simulink model "SpeedgoatCANOpen2Buses100us"  (R2018b)
settings: Solver=ode8  StartTime=0.0  StopTime=inf  FixedStep=0.0001  RelTol=1e-3  EnableMultiTasking=on
undefined symbols (not defined in the file or in its folder): DiscIntNeverNeededParam
libraries: slrtlib x6, speedgoatlib_IO691 x5, simulink x3, dspstat3 x2
(part 2 of 2)

== system SpeedgoatCANOpen2Buses100us/Speedgoat_TPDOs/CAN Bus Communication/CANOpen Slave Protocol Stack - CAN Bus #2 (B) ==
  C Caller : CCaller  FunctionName=CANOpenSlave_ProcessStack_APT  PortSpecificationStruct="%)30     .    ( D   8    (     @         %    \"     8    !     0         %  0 \"0    $    V    07)G3F%M90  4&]R=$YA;64 4V-O<&4     26YD97@     5'EP90      4VEZ90         .    ,     8    (    !          %    \"     $    $     0         0  0 <GA)1 X    P    !@    @    $          4    (     0    0    !         !  ! !R>$E$#@   #@    &    \"     0         !0    @    !    !0    $         $     4   !);G ...(+2763 chars)"
  CAN RX Wrapper : Subsystem
  CAN TX Wrapper : Subsystem
  wires:
  CAN RX Wrapper/3(DATA) -> C Caller/3
  C Caller/3 -> CAN TX Wrapper/3(DATA)
  CAN RX Wrapper/2(DLC) -> C Caller/2
  C Caller/1 -> CAN TX Wrapper/1(ID)
  CAN RX Wrapper/1(ID) -> C Caller/1
  C Caller/2 -> CAN TX Wrapper/2(DLC), CAN TX Wrapper/Enable

== system SpeedgoatCANOpen2Buses100us/Trike Application Layer/System_Control/BrakeControl ==
  Brake control [%] : Inport
  Amp2mAmp : Gain  Gain=1000
  Data Type Conversion : DataTypeConversion  OutDataTypeStr=uint16
  Gain1 : Gain  Gain=12.7
  Gain2 : Gain  Gain=-1
  Gain3 : Gain  Gain=0.00015625
  Saturation : Saturate  UpperLimit=0  LowerLimit=-1
  Saturation1 : Saturate  UpperLimit=10000  LowerLimit=3600
  Sum : Sum  Inputs=|+-
  offset : Constant  Value=3600
  Br CurrentRef [mA] : Outport
  wires:
  Saturation/1 -> Gain1/1
  Gain1/1 -> Amp2mAmp/1
  Brake control [%]/1 -> Data Type Conversion/1
  Gain2/1 -> Saturation/1
  Amp2mAmp/1 -> Br CurrentRef [mA]/1  "Br CurrentRef"
  Sum/1 -> Gain3/1
  offset/1 -> Sum/2
  Gain3/1 -> Gain2/1  "br_percent"
  Data Type Conversion/1 -> Saturation1/1
  Saturation1/1 -> Sum/1

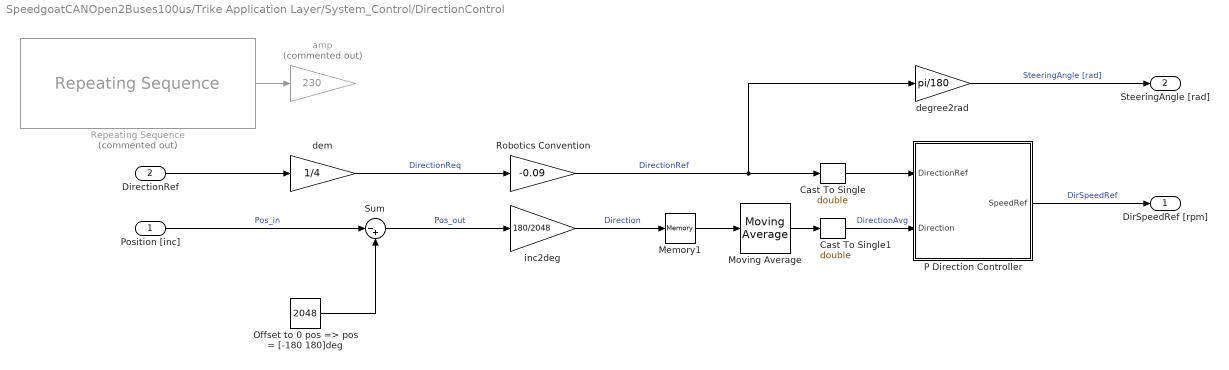
== system SpeedgoatCANOpen2Buses100us/Trike Application Layer/System_Control/DirectionControl ==
  Position [inc] : Inport
  DirectionRef : Inport  Port=2
  Cast To Single : DataTypeConversion  OutDataTypeStr=double
  Cast To Single1 : DataTypeConversion  OutDataTypeStr=double
  Memory1 : Memory  InheritSampleTime=on
  Moving Average : dspstat3/Moving Average  Method=Sliding window  ForgettingFactorPort=off  SpecifyWindowLength=on  WindowLength=1  ForgettingFactor=0.9  SimulateUsing=Code generation
  Offset to 0 pos => pos = [-180 180]deg : Constant  Value=2048
  P Direction Controller : MATLAB Function  TreatAsAtomicUnit=on  SystemSampleTime=5e-3
  Repeating Sequence : simulink/Sources/Repeating Sequence  Commented=on  rep_seq_t=[0 3 3.01 6 6.01 9 9.01 12]*5  rep_seq_y=[1 1 0 0 -1 -1 0 0]
  Robotics Convention : Gain  Gain=-0.09
  Sum : Sum  Inputs=|-+
  amp : Gain  Commented=on  Gain=230
  degree2rad : Gain  Gain=pi/180
  dem : Gain  Gain=1/4
  inc2deg : Gain  Gain=180/2048
  DirSpeedRef [rpm] : Outport
  SteeringAngle [rad] : Outport  Port=2
  wires:
  Memory1/1 -> Moving Average/1
  degree2rad/1 -> SteeringAngle [rad]/1  "SteeringAngle [rad]"
  inc2deg/1 -> Memory1/1  "Direction"
  DirectionRef/1 -> dem/1
  P Direction Controller/1(SpeedRef) -> DirSpeedRef [rpm]/1  "DirSpeedRef"
  Robotics Convention/1 -> Cast To Single/1, degree2rad/1  "DirectionRef"
  Cast To Single/1 -> P Direction Controller/1(DirectionRef)
  Cast To Single1/1 -> P Direction Controller/2(Direction)  "DirectionAvg"
  Position [inc]/1 -> Sum/1  "Pos_in"
  Sum/1 -> inc2deg/1  "Pos_out"
  Offset to 0 pos => pos = [-180 180]deg/1 -> Sum/2
  Moving Average/1 -> Cast To Single1/1
  Repeating Sequence/1 -> amp/1
  dem/1 -> Robotics Convention/1  "DirectionReq"

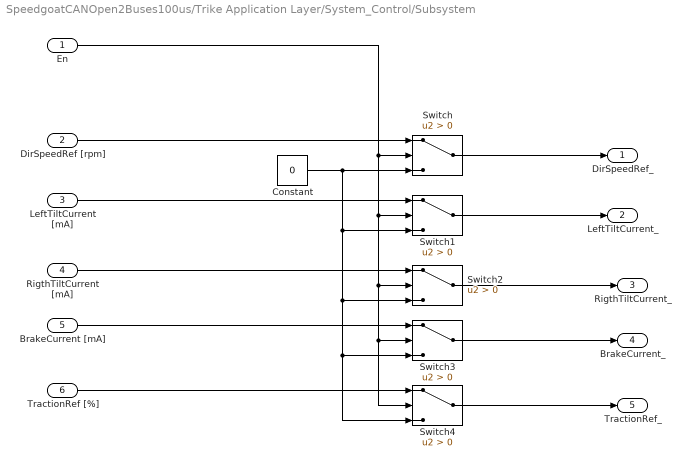
== system SpeedgoatCANOpen2Buses100us/Trike Application Layer/System_Control/Subsystem ==
  En : Inport
  DirSpeedRef [rpm] : Inport  Port=2
  LeftTiltCurrent [mA] : Inport  Port=3
  RigthTiltCurrent [mA] : Inport  Port=4
  BrakeCurrent [mA] : Inport  Port=5
  TractionRef [%] : Inport  Port=6
  Constant : Constant  Value=0
  Switch{,1..4} (5 alike) : Switch  Criteria=u2 > Threshold
  DirSpeedRef_ : Outport
  LeftTiltCurrent_ : Outport  Port=2
  RigthTiltCurrent_ : Outport  Port=3
  BrakeCurrent_ : Outport  Port=4
  TractionRef_ : Outport  Port=5
  wires:
  TractionRef [%]/1 -> Switch4/1
  Switch1/1 -> LeftTiltCurrent_/1
  Switch2/1 -> RigthTiltCurrent_/1
  En/1 -> Switch1/2, Switch2/2, Switch3/2, Switch4/2, Switch/2
  DirSpeedRef [rpm]/1 -> Switch/1
  LeftTiltCurrent [mA]/1 -> Switch1/1
  Constant/1 -> Switch3/3, Switch4/3, Switch2/3, Switch1/3, Switch/3
  Switch/1 -> DirSpeedRef_/1
  BrakeCurrent [mA]/1 -> Switch3/1
  Switch3/1 -> BrakeCurrent_/1
  Switch4/1 -> TractionRef_/1
  RigthTiltCurrent [mA]/1 -> Switch2/1

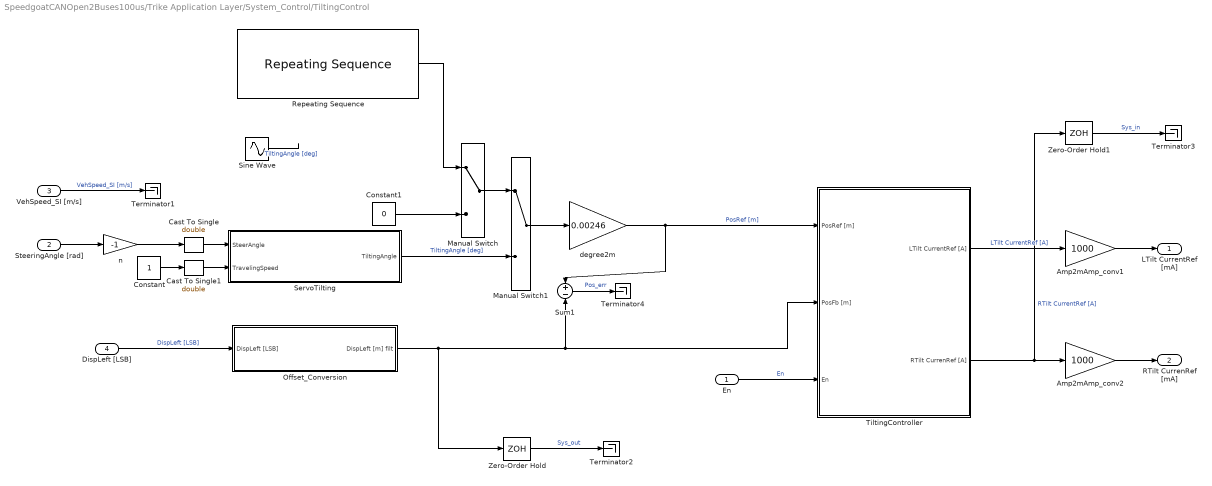
== system SpeedgoatCANOpen2Buses100us/Trike Application Layer/System_Control/TiltingControl ==
  En : Inport
  SteeringAngle [rad] : Inport  Port=2
  VehSpeed_SI [m/s] : Inport  Port=3
  DispLeft [LSB] : Inport  Port=4
  Amp2mAmp_conv1 : Gain  Gain=1000
  Amp2mAmp_conv2 : Gain  Gain=1000
  Cast To Single : DataTypeConversion  OutDataTypeStr=double
  Cast To Single1 : DataTypeConversion  OutDataTypeStr=double
  Constant : Constant
  Constant1 : Constant  Value=0
  Manual Switch : ManualSwitch
  Manual Switch1 : ManualSwitch
  Offset_Conversion : Subsystem
  Repeating Sequence : simulink/Sources/Repeating Sequence  rep_seq_t=[0 3 3.01 6 6.01 9 9.01 12]*5  rep_seq_y=[1 1 0 0 -1 -1 0 0]*2
  ServoTilting : MATLAB Function  TreatAsAtomicUnit=on
      settings: MinAlgLoopOccurrences=on
  Sine Wave : Sin  Frequency=0.5  SampleTime=0
  Sum1 : Sum  Inputs=+|-
  Terminator{1..4} (4 alike) : Terminator
  TiltingController : Subsystem  VariantControlMode=Label  Variant=on  VariantControl=Variant1  LabelModeActiveChoice=V1  PropagateVariantConditions=on
  Zero-Order Hold : ZeroOrderHold  SampleTime=0.001
  Zero-Order Hold1 : ZeroOrderHold  SampleTime=0.001
  degree2m : Gain  Gain=0.00246
  n : Gain  Gain=-1
  LTilt CurrentRef [mA] : Outport
  RTilt CurrenRef [mA] : Outport  Port=2
  wires:
  SteeringAngle [rad]/1 -> n/1
  Constant/1 -> Cast To Single1/1
  Cast To Single/1 -> ServoTilting/1(SteerAngle)
  Cast To Single1/1 -> ServoTilting/2(TravelingSpeed)
  Amp2mAmp_conv1/1 -> LTilt CurrentRef [mA]/1
  Amp2mAmp_conv2/1 -> RTilt CurrenRef [mA]/1
  VehSpeed_SI [m/s]/1 -> Terminator1/1  "VehSpeed_SI [m/s]"
  Constant1/1 -> Manual Switch/2
  ServoTilting/1(TiltingAngle) -> Manual Switch1/2  "TiltingAngle [deg]"
  Manual Switch/1 -> Manual Switch1/1
  Manual Switch1/1 -> degree2m/1
  n/1 -> Cast To Single/1
  degree2m/1 -> Sum1/1, TiltingController/1("PosRef [m] ")  "PosRef [m]"
  Sine Wave/1 -> ?  "TiltingAngle [deg]"
  En/1 -> TiltingController/3("En ")  "En"
  Sum1/1 -> Terminator4/1  "Pos_err"
  TiltingController/1(" LTilt CurrentRef [A]") -> Amp2mAmp_conv1/1  "LTilt CurrentRef [A]"
  TiltingController/2(" RTilt CurrenRef [A]") -> Zero-Order Hold1/1, Amp2mAmp_conv2/1  "RTilt CurrentRef [A]"
  Offset_Conversion/1(DispLeft [m] filt) -> Zero-Order Hold/1, TiltingController/2(PosFb [m]), Sum1/2
  DispLeft [LSB]/1 -> Offset_Conversion/1(DispLeft [LSB])  "DispLeft [LSB]"
  Zero-Order Hold/1 -> Terminator2/1  "Sys_out"
  Zero-Order Hold1/1 -> Terminator3/1  "Sys_in"
  Repeating Sequence/1 -> Manual Switch/1

== system SpeedgoatCANOpen2Buses100us/Trike Application Layer/System_Control/TractionControl ==
  Traction Torque [%] : Inport
  SpeedRear_Fb : Inport  Port=2
  Abs : Abs
  Gain1 : Gain  Gain=1/10
  Gain2 : Gain  Gain=pi/30
  Terminator1 : Terminator
  WheelRadius : Gain  Gain=0.25
  m/s2Km/h : Gain  Gain=3.6
  VehSpeed_SI [m/s] : Outport
  TractionRef [%] : Outport  Port=2
  wires:
  Traction Torque [%]/1 -> Gain1/1
  Abs/1 -> TractionRef [%]/1  "TractionRef"
  WheelRadius/1 -> m/s2Km/h/1, VehSpeed_SI [m/s]/1  "VehSpeed_SI"
  SpeedRear_Fb/1 -> Gain2/1
  Gain2/1 -> WheelRadius/1  "SpeedRear_SI"
  m/s2Km/h/1 -> Terminator1/1  "VehSpeed_Km/h"
  Gain1/1 -> Abs/1

== system SpeedgoatCANOpen2Buses100us/Trike Application Layer/System_Init/Brakes_DunkMotor_Init ==
  Joystick_ButtonStatus : Inport
  DunkD_RPDOs : Inport  Port=2  OutDataTypeStr=Bus: Dunk_RPDOs
  Bus Creator : BusCreator  Inputs=4  OutDataTypeStr=Bus: Dunk_Init_TPDOs
  Bus Selector1 : BusSelector  OutputSignals=DunkD_ActualVelocity
  Cast To Single{,1..3} (4 alike) : DataTypeConversion  OutDataTypeStr=uint8
  Constant : Constant  OutDataTypeStr=single
  DunkD_Brake_Init_CurrentMode : Stateflow chart  TreatAsAtomicUnit=on
  Brakes Motor : Outport  OutDataTypeStr=Bus: Dunk_Init_TPDOs
  Brake InitStatus : Outport  Port=2
  wires:
  DunkD_RPDOs/1 -> Bus Selector1/1
  Bus Creator/1 -> Brakes Motor/1
  Cast To Single1/1 -> Bus Creator/1  "ClearError"
  Cast To Single/1 -> Bus Creator/2  "DeviceMode"
  Cast To Single2/1 -> Bus Creator/3  "BrakeCtrl"
  Cast To Single3/1 -> Bus Creator/4  "PowerEnable"
  DunkD_Brake_Init_CurrentMode/5(InitStatus) -> Brake InitStatus/1
  DunkD_Brake_Init_CurrentMode/1(ClearError) -> Cast To Single1/1
  Joystick_ButtonStatus/1 -> DunkD_Brake_Init_CurrentMode/1(ButtonStatus)
  DunkD_Brake_Init_CurrentMode/2(DeviceMode) -> Cast To Single/1
  DunkD_Brake_Init_CurrentMode/3(BrakeCtrl) -> Cast To Single2/1
  DunkD_Brake_Init_CurrentMode/4(PowerEnable) -> Cast To Single3/1
  Constant/1 -> DunkD_Brake_Init_CurrentMode/2(ReadError)

== system SpeedgoatCANOpen2Buses100us/Trike Application Layer/System_Init/Steering_DunkMotor_Init ==
  Joystick_ButtonStatus : Inport
  DunkA_RPDOs : Inport  Port=2  OutDataTypeStr=Bus: Dunk_RPDOs
  Bus Creator : BusCreator  Inputs=4  OutDataTypeStr=Bus: Dunk_Init_TPDOs
  Bus Selector1 : BusSelector  OutputSignals=DunkA_ActualVelocity
  Cast To Single{,1..3} (4 alike) : DataTypeConversion  OutDataTypeStr=uint8
  Constant : Constant  OutDataTypeStr=single
  DunkA_Steering_Init_SpeedMode : Stateflow chart  TreatAsAtomicUnit=on
  Steering Motor : Outport  OutDataTypeStr=Bus: Dunk_Init_TPDOs
  Steering InitStatus : Outport  Port=2
  wires:
  Bus Creator/1 -> Steering Motor/1
  DunkA_RPDOs/1 -> Bus Selector1/1
  DunkA_Steering_Init_SpeedMode/1(ClearError) -> Cast To Single1/1
  DunkA_Steering_Init_SpeedMode/2(DeviceMode) -> Cast To Single/1
  DunkA_Steering_Init_SpeedMode/3(BrakeCtrl) -> Cast To Single2/1
  DunkA_Steering_Init_SpeedMode/4(PowerEnable) -> Cast To Single3/1
  Joystick_ButtonStatus/1 -> DunkA_Steering_Init_SpeedMode/1(ButtonStatus)
  Constant/1 -> DunkA_Steering_Init_SpeedMode/2(ReadError)
  Cast To Single1/1 -> Bus Creator/1  "ClearError"
  Cast To Single/1 -> Bus Creator/2  "DeviceMode"
  Cast To Single2/1 -> Bus Creator/3  "BrakeCtrl"
  Cast To Single3/1 -> Bus Creator/4  "PowerEnable"
  DunkA_Steering_Init_SpeedMode/5(InitStatus) -> Steering InitStatus/1

== system SpeedgoatCANOpen2Buses100us/Trike Application Layer/System_Init/Subsystem ==
  Steering InitStatus : Inport
  TiltLeft InitStatus : Inport  Port=2
  TiltRight InitStatus : Inport  Port=3
  Brake InitStatus : Inport  Port=4
  MiniMaster_Enable : Inport  Port=5
  Compare To Constant : simulink/Logic and Bit Operations/Compare To Constant  relop===  const=5  OutDataTypeStr=boolean
  Sum : Sum  Inputs=+++++
  EnableControl : Outport
  wires:
  Sum/1 -> Compare To Constant/1
  Brake InitStatus/1 -> Sum/4  "Brake_InitStatus"
  Steering InitStatus/1 -> Sum/1  "Steering_InitStatus"
  TiltRight InitStatus/1 -> Sum/3  "TiltRight_InitStatus"
  TiltLeft InitStatus/1 -> Sum/2  "TiltLeft_InitStatus"
  MiniMaster_Enable/1 -> Sum/5  "MiniMaster_Enable"
  Compare To Constant/1 -> EnableControl/1  "EnableControl"

== system SpeedgoatCANOpen2Buses100us/Trike Application Layer/System_Init/TiltingLeft_DunkMotor_Init ==
  Joystick_ButtonStatus : Inport
  DunkB_RPDOs : Inport  Port=2  OutDataTypeStr=Bus: Dunk_RPDOs
  Bus Creator : BusCreator  Inputs=4  OutDataTypeStr=Bus: Dunk_Init_TPDOs
  Bus Selector1 : BusSelector  OutputSignals=DunkB_ActualVelocity
  Cast To Single{,1..3} (4 alike) : DataTypeConversion  OutDataTypeStr=uint8
  Constant : Constant  OutDataTypeStr=single
  DunkB_TiltLeft_Init_CurrentMode : Stateflow chart  TreatAsAtomicUnit=on
  TiltLeft Motor : Outport  OutDataTypeStr=Bus: Dunk_Init_TPDOs
  TiltLeft InitStatus : Outport  Port=2
  wires:
  DunkB_RPDOs/1 -> Bus Selector1/1
  Bus Creator/1 -> TiltLeft Motor/1
  DunkB_TiltLeft_Init_CurrentMode/5(InitStatus) -> TiltLeft InitStatus/1
  Cast To Single/1 -> Bus Creator/2  "DeviceMode"
  Constant/1 -> DunkB_TiltLeft_Init_CurrentMode/2(ReadError)
  Cast To Single2/1 -> Bus Creator/3  "BrakeCtrl"
  DunkB_TiltLeft_Init_CurrentMode/4(PowerEnable) -> Cast To Single3/1
  DunkB_TiltLeft_Init_CurrentMode/3(BrakeCtrl) -> Cast To Single2/1
  Cast To Single3/1 -> Bus Creator/4  "PowerEnable"
  DunkB_TiltLeft_Init_CurrentMode/2(DeviceMode) -> Cast To Single/1
  Cast To Single1/1 -> Bus Creator/1  "ClearError"
  DunkB_TiltLeft_Init_CurrentMode/1(ClearError) -> Cast To Single1/1
  Joystick_ButtonStatus/1 -> DunkB_TiltLeft_Init_CurrentMode/1(ButtonStatus)

== system SpeedgoatCANOpen2Buses100us/Trike Application Layer/System_Init/TiltingRight_DunkMotor_Init ==
  Joystick_ButtonStatus : Inport
  DunkC_RPDOs : Inport  Port=2  OutDataTypeStr=Bus: Dunk_RPDOs
  Bus Creator : BusCreator  Inputs=4  OutDataTypeStr=Bus: Dunk_Init_TPDOs
  Bus Selector1 : BusSelector  OutputSignals=DunkC_ActualVelocity
  Cast To Single{,1..3} (4 alike) : DataTypeConversion  OutDataTypeStr=uint8
  Constant : Constant  OutDataTypeStr=single
  DunkC_TiltRight_Init_CurrentMode : Stateflow chart  TreatAsAtomicUnit=on
  TiltRight Motor : Outport  OutDataTypeStr=Bus: Dunk_Init_TPDOs
  TiltRight InitStatus : Outport  Port=2
  wires:
  Bus Creator/1 -> TiltRight Motor/1
  DunkC_RPDOs/1 -> Bus Selector1/1
  Cast To Single1/1 -> Bus Creator/1  "ClearError"
  Cast To Single/1 -> Bus Creator/2  "DeviceMode"
  Cast To Single2/1 -> Bus Creator/3  "BrakeCtrl"
  Cast To Single3/1 -> Bus Creator/4  "PowerEnable"
  DunkC_TiltRight_Init_CurrentMode/5(InitStatus) -> TiltRight InitStatus/1
  DunkC_TiltRight_Init_CurrentMode/1(ClearError) -> Cast To Single1/1
  Joystick_ButtonStatus/1 -> DunkC_TiltRight_Init_CurrentMode/1(ButtonStatus)
  DunkC_TiltRight_Init_CurrentMode/2(DeviceMode) -> Cast To Single/1
  DunkC_TiltRight_Init_CurrentMode/3(BrakeCtrl) -> Cast To Single2/1
  DunkC_TiltRight_Init_CurrentMode/4(PowerEnable) -> Cast To Single3/1
  Constant/1 -> DunkC_TiltRight_Init_CurrentMode/2(ReadError)

== system SpeedgoatCANOpen2Buses100us/Speedgoat_TPDOs/CAN Bus Communication/CANOpen Slave Protocol Stack - CAN Bus #1 (A)/CAN RX Wrapper ==
  CAN Read : speedgoatlib_IO691/CAN Read  id=1  ts=Ts  channel=1  messageType=RAW  canType=CAN (HS)  initValues=[691 1 0.0001 0 2 1]
      settings: SourceProductName=Simulink Real-Time: Speedgoat Library
  Constant : Constant  Commented=on  Value=0  OutDataTypeStr=Inherit: Inherit via back propagation
  Switch : Switch  Criteria=u2 > Threshold
  Terminator : Terminator
  Terminator1 : Terminator
  ID : Outport
  DLC : Outport  Port=2
  DATA : Outport  Port=3
  wires:
  CAN Read/4 -> Switch/3
  CAN Read/5 -> Terminator1/1
  Switch/1 -> DLC/1
  CAN Read/2 -> ID/1
  CAN Read/3 -> Switch/2
  CAN Read/6 -> DATA/1
  Constant/1 -> Switch/1
  CAN Read/1 -> Terminator/1

== system SpeedgoatCANOpen2Buses100us/Speedgoat_TPDOs/CAN Bus Communication/CANOpen Slave Protocol Stack - CAN Bus #1 (A)/CAN TX Wrapper ==
  ID : Inport
  DLC : Inport  Port=2
  DATA : Inport  Port=3
  Enable : EnablePort
  CAN Write : speedgoatlib_IO691/CAN Write  id=1  ts=Ts  channel=1  messageType=RAW  enableStatusPort=off  canType=CAN (HS)  initValues=[691 1 0.0001 0 2 1 0]
      settings: SourceProductName=Simulink Real-Time: Speedgoat Library
  Constant : Constant  Value=0  OutDataTypeStr=Inherit: Inherit via back propagation
  wires:
  ID/1 -> CAN Write/1
  DATA/1 -> CAN Write/4
  DLC/1 -> CAN Write/3
  Constant/1 -> CAN Write/2

== system SpeedgoatCANOpen2Buses100us/Speedgoat_TPDOs/CAN Bus Communication/CANOpen Slave Protocol Stack - CAN Bus #2 (B)/CAN RX Wrapper ==
  CAN Read : speedgoatlib_IO691/CAN Read  id=1  ts=Ts  channel=2  messageType=RAW  canType=CAN (HS)  initValues=[691 1 0.0001 1 2 1]
      settings: SourceProductName=Simulink Real-Time: Speedgoat Library
  Constant : Constant  Commented=on  Value=0  OutDataTypeStr=Inherit: Inherit via back propagation
  Switch : Switch  Criteria=u2 > Threshold
  Terminator : Terminator
  Terminator1 : Terminator
  ID : Outport
  DLC : Outport  Port=2
  DATA : Outport  Port=3
  wires:
  CAN Read/1 -> Terminator/1
  Constant/1 -> Switch/1
  CAN Read/6 -> DATA/1
  CAN Read/3 -> Switch/2
  CAN Read/2 -> ID/1
  Switch/1 -> DLC/1
  CAN Read/5 -> Terminator1/1
  CAN Read/4 -> Switch/3

== system SpeedgoatCANOpen2Buses100us/Speedgoat_TPDOs/CAN Bus Communication/CANOpen Slave Protocol Stack - CAN Bus #2 (B)/CAN TX Wrapper ==
  ID : Inport
  DLC : Inport  Port=2
  DATA : Inport  Port=3
  Enable : EnablePort
  CAN Write : speedgoatlib_IO691/CAN Write  id=1  ts=Ts  channel=2  messageType=RAW  enableStatusPort=off  canType=CAN (HS)  initValues=[691 1 0.0001 1 2 1 0]
      settings: SourceProductName=Simulink Real-Time: Speedgoat Library
  Constant : Constant  Value=0  OutDataTypeStr=Inherit: Inherit via back propagation
  wires:
  Constant/1 -> CAN Write/2
  DLC/1 -> CAN Write/3
  DATA/1 -> CAN Write/4
  ID/1 -> CAN Write/1

== system SpeedgoatCANOpen2Buses100us/Trike Application Layer/System_Control/TiltingControl/Offset_Conversion ==
  DispLeft [LSB] : Inport
  Discrete Filter : DiscreteFilter  Numerator=[0.0201 0.0402 0.0201]  Denominator=[1 -1.561 0.6414]  SampleTime=0.005
  LSB2Volt : Gain  Gain=5/16380
  Memory1 : Memory  InheritSampleTime=on
  "Offset for 0 deg (3.5064V -> 57.02mm)" : Constant  Value=3.5064
  Sum : Sum  Inputs=|+-
  Volt2meter : Gain  Gain=0.076/5
  DispLeft [m] filt : Outport
  wires:
  Volt2meter/1 -> Memory1/1, Discrete Filter/1  "DispLeft [m]"
  "Offset for 0 deg (3.5064V -> 57.02mm)"/1 -> Sum/2
  Sum/1 -> Volt2meter/1  "DispLeftOffset [Volt]"
  LSB2Volt/1 -> Sum/1  "DispLeft [Volt]"
  Discrete Filter/1 -> ?
  Memory1/1 -> DispLeft [m] filt/1  "DispLeft [m] filt"
  DispLeft [LSB]/1 -> LSB2Volt/1

== system SpeedgoatCANOpen2Buses100us/Trike Application Layer/System_Control/TiltingControl/TiltingController ==
  "PosRef [m] " : Inport
  PosFb [m] : Inport  Port=2
  "En " : Inport  Port=3
  PID_Adaptiv_V2 : Subsystem  VariantControl=V0
  PID_Clasic_V1 : Subsystem  VariantControl=V1
  PID_Incremental_V1 : Subsystem  VariantControl=V2
  PID_Incremental_V2 : Subsystem  VariantControl=V3
  " LTilt CurrentRef [A]" : Outport
  " RTilt CurrenRef [A]" : Outport  Port=2

== system SpeedgoatCANOpen2Buses100us/Trike Application Layer/System_Control/TiltingControl/TiltingController/PID_Adaptiv_V2 ==
  PosRef [m] : Inport
  PosFb [m] : Inport  Port=2
  En : Inport  Port=3
  PID_ctrl : Subsystem  mask{Kp=800, Ki=400, Kd=0, Ts=0.001, N=1, FF_En=1, Req_lim=10}
      mask prompts: N "FilterOrder"; FF_En "FeedForward En"; Req_lim "Req_sat"
  " LTilt CurrentRef [A]" : Outport
  " RTilt CurrenRef [A]" : Outport  Port=2
  wires:
  PosRef [m]/1 -> PID_ctrl/1(PosRef)
  PosFb [m]/1 -> PID_ctrl/2(PosFb)
  PID_ctrl/1(LTilt CurrentRef [A]) -> " LTilt CurrentRef [A]"/1  "LTilt CurrentRef"
  PID_ctrl/2(RTilt CurrentRef [A]) -> " RTilt CurrenRef [A]"/1  "RTilt CurrenRef"
  En/1 -> PID_ctrl/3(En)

== system SpeedgoatCANOpen2Buses100us/Trike Application Layer/System_Control/TiltingControl/TiltingController/PID_Clasic_V1 ==
  PosRef [m] : Inport
  PosFb [m] : Inport  Port=2
  En : Inport  Port=3
  PID_ctrl : Subsystem  mask{Kp=800, Ki=400, Kd=0, Ts=0.001, N=1, FF_En=1, Req_lim=10}
      mask prompts: N "FilterOrder"; FF_En "FeedForward En"; Req_lim "Req_sat"
  " LTilt CurrentRef [A]" : Outport
  " RTilt CurrenRef [A]" : Outport  Port=2
  wires:
  En/1 -> PID_ctrl/3(En)
  PID_ctrl/2(RTilt CurrentRef [A]) -> " RTilt CurrenRef [A]"/1  "RTilt CurrenRef"
  PID_ctrl/1(LTilt CurrentRef [A]) -> " LTilt CurrentRef [A]"/1  "LTilt CurrentRef"
  PosFb [m]/1 -> PID_ctrl/2(PosFb)
  PosRef [m]/1 -> PID_ctrl/1(PosRef)

== system SpeedgoatCANOpen2Buses100us/Trike Application Layer/System_Control/TiltingControl/TiltingController/PID_Incremental_V1 ==
  PosRef [m] : Inport
  PosFb [m] : Inport  Port=2
  En : Inport  Port=3
  PI_incremental Tilting Controller : MATLAB Function  TreatAsAtomicUnit=on  SystemSampleTime=5e-3
  Terminator1 : Terminator
  Terminator2 : Terminator
  Terminator7 : Terminator
  " LTilt CurrentRef [A]" : Outport
  " RTilt CurrenRef [A]" : Outport  Port=2
  wires:
  En/1 -> PI_incremental Tilting Controller/3(En)
  PI_incremental Tilting Controller/2(RTiltCurrRef) -> " RTilt CurrenRef [A]"/1  "RTilt CurrenRef"
  PI_incremental Tilting Controller/1(LTiltCurrRef) -> " LTilt CurrentRef [A]"/1  "LTilt CurrentRef"
  PosFb [m]/1 -> PI_incremental Tilting Controller/2(Pos)
  PosRef [m]/1 -> PI_incremental Tilting Controller/1(PosRef)
  PI_incremental Tilting Controller/3(up) -> Terminator7/1  "up"
  PI_incremental Tilting Controller/4(ui) -> Terminator1/1  "ui"
  PI_incremental Tilting Controller/5(ud) -> Terminator2/1  "ud"

== system SpeedgoatCANOpen2Buses100us/Trike Application Layer/System_Control/TiltingControl/TiltingController/PID_Incremental_V2 ==
  PosRef [m] : Inport
  PosFb [m] : Inport  Port=2
  En : Inport  Port=3
  MATLAB Function : MATLAB Function  TreatAsAtomicUnit=on  SystemSampleTime=0.005
  Terminator1 : Terminator
  Terminator7 : Terminator
  " LTilt CurrentRef [A]" : Outport
  " RTilt CurrenRef [A]" : Outport  Port=2
  wires:
  PosRef [m]/1 -> MATLAB Function/1(PosRef)
  PosFb [m]/1 -> MATLAB Function/2(Pos)
  MATLAB Function/1(LTiltCurrRef) -> " LTilt CurrentRef [A]"/1  "LTilt CurrentRef"
  MATLAB Function/3(c1) -> Terminator7/1  "c1"
  MATLAB Function/2(RTiltCurrRef) -> " RTilt CurrenRef [A]"/1  "RTilt CurrenRef"
  En/1 -> MATLAB Function/3(En)
  MATLAB Function/4(c2) -> Terminator1/1  "c2"

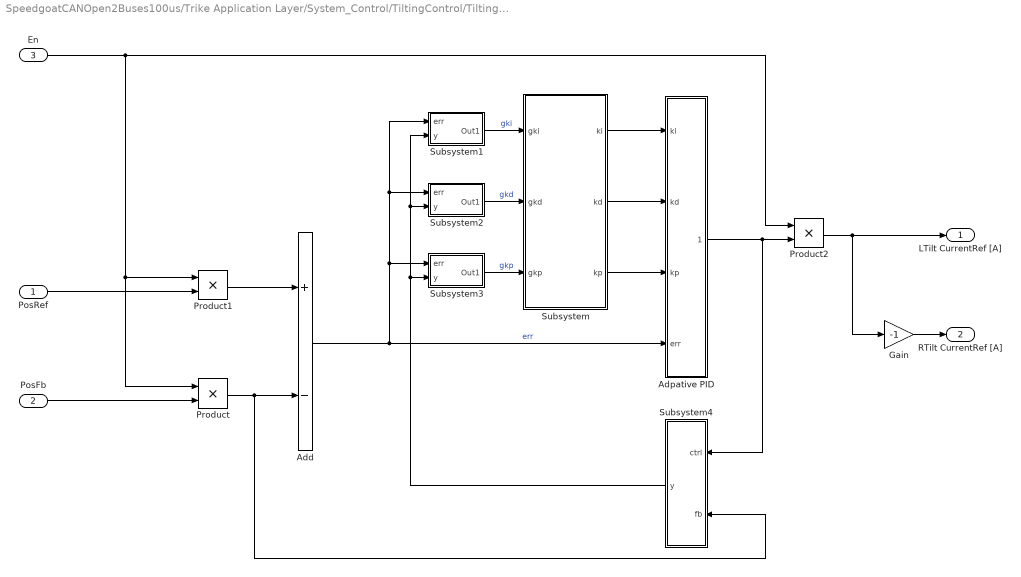
== system SpeedgoatCANOpen2Buses100us/Trike Application Layer/System_Control/TiltingControl/TiltingController/PID_Adaptiv_V2/PID_ctrl ==
  PosRef : Inport
  PosFb : Inport  Port=2
  En : Inport  Port=3
  Add : Sum  Inputs=+-
  Adpative PID : Subsystem
  Gain : Gain  Gain=-1
  Product : Product
  Product1 : Product
  Product2 : Product
  Subsystem : Subsystem
  Subsystem1 : Subsystem
  Subsystem2 : Subsystem
  Subsystem3 : Subsystem
  Subsystem4 : Subsystem
  LTilt CurrentRef [A] : Outport  VectorParamsAs1DForOutWhenUnconnected=on
  RTilt CurrentRef [A] : Outport  Port=2  VectorParamsAs1DForOutWhenUnconnected=on
  wires:
  Gain/1 -> RTilt CurrentRef [A]/1
  Product2/1 -> LTilt CurrentRef [A]/1, Gain/1
  PosRef/1 -> Product1/2
  En/1 -> Product1/1, Product/1, Product2/1
  PosFb/1 -> Product/2
  Subsystem1/1(Out1) -> Subsystem/1(gki)  "gki"
  Subsystem/2(kd) -> Adpative PID/2(kd)
  Subsystem3/1(Out1) -> Subsystem/3(gkp)  "gkp"
  Subsystem/1(ki) -> Adpative PID/1(ki)
  Subsystem/3(kp) -> Adpative PID/3(kp)
  Subsystem2/1(Out1) -> Subsystem/2(gkd)  "gkd"
  Subsystem4/1(y) -> Subsystem3/2(y), Subsystem2/2(y), Subsystem1/2(y)
  Adpative PID/1(ctrl) -> Subsystem4/1(ctrl), Product2/2
  Add/1 -> Subsystem1/1(err), Subsystem2/1(err), Subsystem3/1(err), Adpative PID/4(err)  "err"
  Product1/1 -> Add/1
  Product/1 -> Subsystem4/2(fb), Add/2

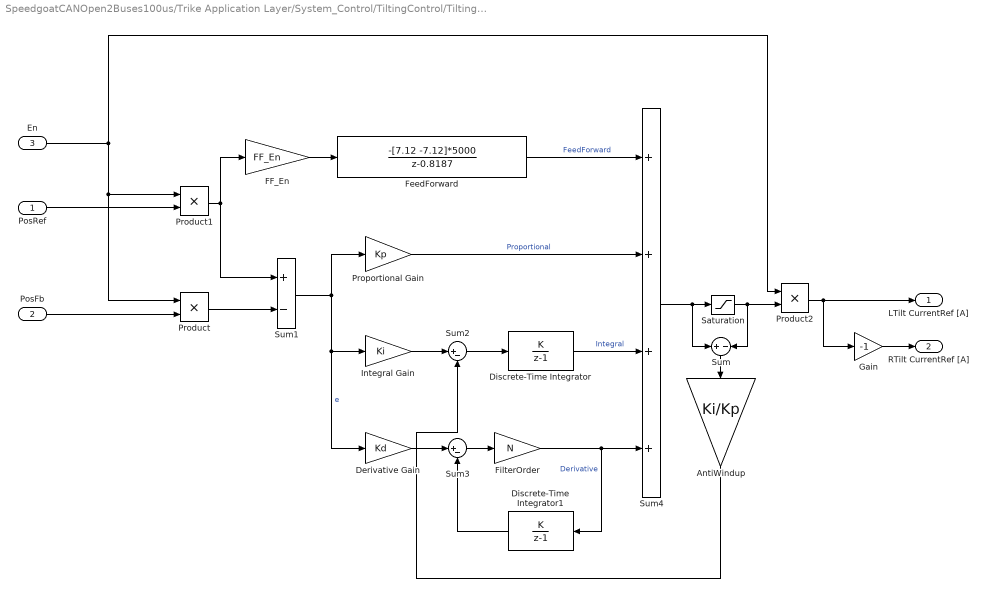
== system SpeedgoatCANOpen2Buses100us/Trike Application Layer/System_Control/TiltingControl/TiltingController/PID_Clasic_V1/PID_ctrl ==
  PosRef : Inport
  PosFb : Inport  Port=2
  En : Inport  Port=3
  AntiWindup : Gain  Gain=Ki/Kp  SaturateOnIntegerOverflow=on  OutDataTypeStr=Inherit: Same as input  ParamDataTypeStr=Inherit: Same as input
  Derivative Gain : Gain  Gain=Kd  SaturateOnIntegerOverflow=on  OutDataTypeStr=Inherit: Same as input  ParamDataTypeStr=Inherit: Same as input
  Discrete-Time Integrator : DiscreteIntegrator  IntegratorMethod=Accumulation: Forward Euler  gainval=Ts/5  SampleTime=-1  ICPrevOutput=DiscIntNeverNeededParam  ICPrevScaledInput=DiscIntNeverNeededParam
  Discrete-Time Integrator1 : DiscreteIntegrator  IntegratorMethod=Accumulation: Forward Euler  gainval=Ts/5  SampleTime=-1  ICPrevOutput=DiscIntNeverNeededParam  ICPrevScaledInput=DiscIntNeverNeededParam
  FF_En : Gain  Gain=FF_En  SaturateOnIntegerOverflow=on  OutDataTypeStr=Inherit: Same as input  ParamDataTypeStr=Inherit: Same as input
  FeedForward : DiscreteTransferFcn  Numerator=-[7.12 -7.12]*5000  Denominator=[1 -0.8187]  SampleTime=Ts/5
  FilterOrder : Gain  Gain=N  SaturateOnIntegerOverflow=on  OutDataTypeStr=Inherit: Same as input  ParamDataTypeStr=Inherit: Same as input
  Gain : Gain  Gain=-1
  Integral Gain : Gain  Gain=Ki  SaturateOnIntegerOverflow=on  OutDataTypeStr=Inherit: Same as input  ParamDataTypeStr=Inherit: Same as input
  Product : Product
  Product1 : Product
  Product2 : Product
  Proportional Gain : Gain  Gain=Kp  SaturateOnIntegerOverflow=on  OutDataTypeStr=Inherit: Same as input  ParamDataTypeStr=Inherit: Same as input
  Saturation : Saturate  UpperLimit=Req_lim  LowerLimit=-Req_lim
  Sum : Sum  Inputs=+|-
  Sum1 : Sum  Inputs=+-  SaturateOnIntegerOverflow=on  InputSameDT=on  OutDataTypeStr=Inherit: Same as first input
  Sum2 : Sum  Inputs=|+-
  Sum3 : Sum  Inputs=|+-
  Sum4 : Sum  Inputs=++++  SaturateOnIntegerOverflow=on  InputSameDT=on  OutDataTypeStr=Inherit: Same as first input
  LTilt CurrentRef [A] : Outport  VectorParamsAs1DForOutWhenUnconnected=on
  RTilt CurrentRef [A] : Outport  Port=2  VectorParamsAs1DForOutWhenUnconnected=on
  wires:
  Saturation/1 -> Product2/2, Sum/2
  AntiWindup/1 -> Sum2/2
  Sum2/1 -> Discrete-Time Integrator/1
  Sum4/1 -> Sum/1, Saturation/1
  FeedForward/1 -> Sum4/1  "FeedForward"
  Proportional Gain/1 -> Sum4/2  "Proportional"
  Integral Gain/1 -> Sum2/1
  Sum/1 -> AntiWindup/1
  Discrete-Time Integrator/1 -> Sum4/3  "Integral"
  PosFb/1 -> Product/2
  Product1/1 -> Sum1/1, FF_En/1
  Product/1 -> Sum1/2
  En/1 -> Product2/1, Product/1, Product1/1
  PosRef/1 -> Product1/2
  Product2/1 -> Gain/1, LTilt CurrentRef [A]/1
  Gain/1 -> RTilt CurrentRef [A]/1
  Derivative Gain/1 -> Sum3/1
  Discrete-Time Integrator1/1 -> Sum3/2
  Sum1/1 -> Proportional Gain/1, Derivative Gain/1, Integral Gain/1  "e"
  Sum3/1 -> FilterOrder/1
  FilterOrder/1 -> Sum4/4, Discrete-Time Integrator1/1  "Derivative"
  FF_En/1 -> FeedForward/1

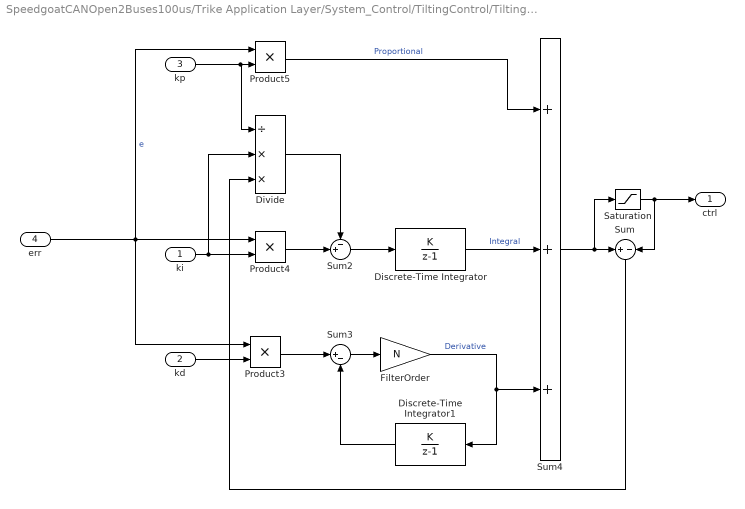
== system SpeedgoatCANOpen2Buses100us/Trike Application Layer/System_Control/TiltingControl/TiltingController/PID_Adaptiv_V2/PID_ctrl/Adpative PID ==
  ki : Inport
  kd : Inport  Port=2
  kp : Inport  Port=3
  err : Inport  Port=4
  Discrete-Time Integrator : DiscreteIntegrator  IntegratorMethod=Accumulation: Forward Euler  gainval=Ts/2  SampleTime=-1  ICPrevOutput=DiscIntNeverNeededParam  ICPrevScaledInput=DiscIntNeverNeededParam
  Discrete-Time Integrator1 : DiscreteIntegrator  IntegratorMethod=Accumulation: Forward Euler  gainval=Ts/2  SampleTime=-1  ICPrevOutput=DiscIntNeverNeededParam  ICPrevScaledInput=DiscIntNeverNeededParam
  Divide : Product  Inputs=/**
  FilterOrder : Gain  Gain=N  SaturateOnIntegerOverflow=on  OutDataTypeStr=Inherit: Same as input  ParamDataTypeStr=Inherit: Same as input
  Product3 : Product
  Product4 : Product
  Product5 : Product
  Saturation : Saturate  UpperLimit=Req_lim  LowerLimit=-Req_lim
  Sum : Sum  Inputs=+|-
  Sum2 : Sum  Inputs=-+|
  Sum3 : Sum  Inputs=|+-
  Sum4 : Sum  Inputs=+++  SaturateOnIntegerOverflow=on  InputSameDT=on  OutDataTypeStr=Inherit: Same as first input
  ctrl : Outport  VectorParamsAs1DForOutWhenUnconnected=on
  wires:
  Discrete-Time Integrator/1 -> Sum4/2  "Integral"
  Discrete-Time Integrator1/1 -> Sum3/2
  Sum/1 -> Divide/3
  Sum2/1 -> Discrete-Time Integrator/1
  Product3/1 -> Sum3/1
  Sum3/1 -> FilterOrder/1
  Product4/1 -> Sum2/2
  FilterOrder/1 -> Sum4/3, Discrete-Time Integrator1/1  "Derivative"
  Product5/1 -> Sum4/1  "Proportional"
  Saturation/1 -> ctrl/1, Sum/2
  err/1 -> Product4/1, Product3/1, Product5/1  "e"
  Sum4/1 -> Saturation/1, Sum/1
  kp/1 -> Divide/1, Product5/2
  ki/1 -> Product4/2, Divide/2
  kd/1 -> Product3/2
  Divide/1 -> Sum2/1

== system SpeedgoatCANOpen2Buses100us/Trike Application Layer/System_Control/TiltingControl/TiltingController/PID_Adaptiv_V2/PID_ctrl/Subsystem ==
  gki : Inport
  gkd : Inport  Port=2
  gkp : Inport  Port=3
  Alpha : Constant  Value=1000
  MATLAB Function : MATLAB Function  TreatAsAtomicUnit=on
  Unit Delay : UnitDelay  InitialCondition=Kp  SampleTime=1e-3
  Unit Delay1 : UnitDelay  InitialCondition=Ki  SampleTime=1e-3
  Unit Delay2 : UnitDelay  InitialCondition=Kd  SampleTime=1e-3
  Unit Delay4 : UnitDelay  SampleTime=1e-3
  Unit Delay5 : UnitDelay  SampleTime=1e-3
  Unit Delay6 : UnitDelay  SampleTime=1e-3
  ki : Outport  VectorParamsAs1DForOutWhenUnconnected=on
  kd : Outport  Port=2  VectorParamsAs1DForOutWhenUnconnected=on
  kp : Outport  Port=3  VectorParamsAs1DForOutWhenUnconnected=on
  wires:
  Unit Delay4/1 -> MATLAB Function/8("gradKp_old ")
  MATLAB Function/2(Kd) -> kd/1, Unit Delay2/1  "kd"
  MATLAB Function/6(gradKd_old) -> Unit Delay6/1
  Unit Delay1/1 -> MATLAB Function/6(Ki_old)
  MATLAB Function/4(gradKp_old) -> Unit Delay4/1
  Alpha/1 -> MATLAB Function/4(alpha)
  MATLAB Function/5(gradKi_old) -> Unit Delay5/1
  MATLAB Function/3(Kp) -> kp/1, Unit Delay/1  "kp"
  Unit Delay6/1 -> MATLAB Function/10("gradKd_old ")
  Unit Delay/1 -> MATLAB Function/5(Kp_old)
  MATLAB Function/1(Ki) -> ki/1, Unit Delay1/1  "ki"
  Unit Delay5/1 -> MATLAB Function/9("gradKi_old ")
  Unit Delay2/1 -> MATLAB Function/7(Kd_old)
  gki/1 -> MATLAB Function/1(gradKi)
  gkd/1 -> MATLAB Function/2(gradKd)
  gkp/1 -> MATLAB Function/3(gradKp)

== system SpeedgoatCANOpen2Buses100us/Trike Application Layer/System_Control/TiltingControl/TiltingController/PID_Adaptiv_V2/PID_ctrl/Subsystem1 ==
  err : Inport
  y : Inport  Port=2
  Discrete-Time Integrator : DiscreteIntegrator  IntegratorMethod=Accumulation: Forward Euler  gainval=0.0001  SampleTime=-1  ICPrevOutput=DiscIntNeverNeededParam  ICPrevScaledInput=DiscIntNeverNeededParam
  Gain : Gain  Gain=-1
  Product : Product
  Product1 : Product
  Out1 : Outport  VectorParamsAs1DForOutWhenUnconnected=on
  wires:
  Discrete-Time Integrator/1 -> Product1/2
  Gain/1 -> Product/1
  Product1/1 -> Out1/1
  Product/1 -> Product1/1
  y/1 -> Product/2
  err/1 -> Discrete-Time Integrator/1, Gain/1

== system SpeedgoatCANOpen2Buses100us/Trike Application Layer/System_Control/TiltingControl/TiltingController/PID_Adaptiv_V2/PID_ctrl/Subsystem2 ==
  err : Inport
  y : Inport  Port=2
  Discrete-Time Integrator1 : DiscreteIntegrator  IntegratorMethod=Accumulation: Forward Euler  gainval=0.0001  SampleTime=-1  ICPrevOutput=DiscIntNeverNeededParam  ICPrevScaledInput=DiscIntNeverNeededParam
  FilterOrder : Gain  SaturateOnIntegerOverflow=on  OutDataTypeStr=Inherit: Same as input  ParamDataTypeStr=Inherit: Same as input
  Gain : Gain  Gain=-1
  Product : Product
  Product1 : Product
  Sum3 : Sum  Inputs=|+-
  Out1 : Outport  VectorParamsAs1DForOutWhenUnconnected=on
  wires:
  y/1 -> Product/2
  Product/1 -> Product1/1
  Product1/1 -> Out1/1
  Gain/1 -> Product/1
  err/1 -> Sum3/1, Gain/1
  Sum3/1 -> FilterOrder/1
  Discrete-Time Integrator1/1 -> Sum3/2
  FilterOrder/1 -> Discrete-Time Integrator1/1, Product1/2

== system SpeedgoatCANOpen2Buses100us/Trike Application Layer/System_Control/TiltingControl/TiltingController/PID_Adaptiv_V2/PID_ctrl/Subsystem3 ==
  err : Inport
  y : Inport  Port=2
  Gain : Gain  Gain=-1
  Product : Product
  Product1 : Product
  Out1 : Outport  VectorParamsAs1DForOutWhenUnconnected=on
  wires:
  Gain/1 -> Product/1
  Product1/1 -> Out1/1
  Product/1 -> Product1/1
  y/1 -> Product/2
  err/1 -> Gain/1, Product1/2

== system SpeedgoatCANOpen2Buses100us/Trike Application Layer/System_Control/TiltingControl/TiltingController/PID_Adaptiv_V2/PID_ctrl/Subsystem4 ==
  ctrl : Inport
  fb : Inport  Port=2
  Constant : Constant  Value=|
      | [0.811661315567532	0.523339604043497
      | 0.781547366351639	0.164018692936968
      | 0.146098503423341	0.879428705628321
      | 0.266102211582170	0.304501614309624
      | 0.397284814093776	0.765244619952808
      | 0.516628753495178	0.186405621841320
      | 0.0862525926601981	0.717804970916536
      | 0.103414091455425	0.420647287190983
      | 0.506698658207659	0.609237422549281
      | 0.269175608561842	0.124471251020265
      | 0.0151134208657587	0.418749009267761
      | 0.873047701593747	0.980270684978551
      | 0.0624305176835148	0.302769416201919
      | 0.0444243510475763	0.430246616185495
      | 0.956127765123271	0.142311041042483
      | 0.549202286331316	0.311122631590002
      | 0.713499976100381	0.159301438083396
      | 0.328775895527325	0.385292704689736
      | 0.649001722373211	0.236663924286235
      | 0.0654762342586071	0.315797884817915]
  Constant2 : Constant  Value="[0.610759087177597\t0.366179666335005\t-0.0584030572951834\t0.209075859992505\t0.584389586358981\t0.349871470561781\t-0.204405272265807\t-0.116182445469499\t0.0642557952818070\t-0.132902026263845\t0.805831183296775\t-0.399691016290584\t0.259161704540015\t0.179474388613012\t-0.0314937390524749\t0.704808744971737\t0.263155510958995\t0.213381634610559\t0.587918070221544\t0.290284501669435]"
  Constant3 : Constant  Value=|
      | [0.818045624381218
      | 0.102878023447675
      | 0.737296135799067
      | 0.382188425410472
      | 0.977505309905872
      | 0.149360203196300
      | 0.641439600546557
      | 0.443497484934195
      | 0.680421925309724
      | 0.859879825832941
      | -0.318689482669828
      | 0.255207188653107
      | 0.313389787503390
      | 0.721063295306122
      | 0.439116073494923
      | -0.219038629148731
      | 0.491813043211072
      | -0.0750940652226708
      | -0.120979967962816
      | 0.00273892356427859]
  Delay : Delay  DelayLength=1  SampleTime=1e-3
  Gain : Gain  Gain=1e-5
  Gain1 : Gain  Gain=1/20
  MATLAB Function1 : MATLAB Function  TreatAsAtomicUnit=on
  Unit Delay3 : UnitDelay  SampleTime=1e-3
  derivativeNN : MATLAB Function  TreatAsAtomicUnit=on
  y : Outport  VectorParamsAs1DForOutWhenUnconnected=on
  wires:
  Gain/1 -> derivativeNN/1(X1)
  derivativeNN/1(dydu) -> MATLAB Function1/1(u)
  Constant2/1 -> derivativeNN/4(Wout)
  Constant/1 -> derivativeNN/3(Win)
  Constant3/1 -> derivativeNN/5(bin)
  Delay/1 -> Gain1/1
  Gain1/1 -> derivativeNN/2(X2)
  MATLAB Function1/1(y) -> Unit Delay3/1
  ctrl/1 -> Gain/1
  Unit Delay3/1 -> y/1
  fb/1 -> Delay/1

== stateflow chart SpeedgoatCANOpen2Buses100us/Trike Application Layer/System_Init/TiltingLeft_DunkMotor_Init/DunkB_TiltLeft_Init_CurrentMode ==
  state Init
    entry:
    ClearError       = 0;
    DeviceMode   = 0;
    BrakeCtrl        = 0;
    PowerEnable = 0;
    aux                 = 0;
    InitStatus        = 0;
  state Clear_Error
    du:
    ClearError = 1;
    aux=aux+1;
    InitStatus = 0;
  state Wait
    en:
    BrakeCtrl = 2;
    aux = 0;
    InitStatus = 0;
  state SetCurrentMode
    du:
    DeviceMode  = 2;
    PowerEnable = 1;
    InitStatus       = 1;
  (default) -> Init
  Init -> Clear_Error : [ButtonStatus == 1 || ReadError ~= 1]
  Wait -> Init [order 3] : [ReadError ~= 1]
  SetCurrentMode -> Init : [ReadError ~= 1]
  Clear_Error -> Wait : [aux>2000]
  Wait -> Wait [order 1] : [ButtonStatus==0 && ReadError == 1]
  Wait -> SetCurrentMode [order 2] : [ButtonStatus==2 && ReadError == 1]
  data: ButtonStatus input single; ClearError output single; DeviceMode output single; BrakeCtrl output single; ReadError input single; aux2 local single; aux local single; PowerEnable output single; InitStatus output single

== stateflow chart SpeedgoatCANOpen2Buses100us/Trike Application Layer/System_Init/TiltingRight_DunkMotor_Init/DunkC_TiltRight_Init_CurrentMode ==
  state Init
    entry:
    ClearError       = 0;
    DeviceMode   = 0;
    BrakeCtrl        = 0;
    PowerEnable = 0;
    aux                 = 0;
    InitStatus        = 0;
  state Clear_Error
    du:
    ClearError = 1;
    aux=aux+1;
    InitStatus = 0;
  state Wait
    en:
    BrakeCtrl = 2;
    aux = 0;
    InitStatus = 0;
  state SetCurrentMode
    du:
    DeviceMode  = 2;
    PowerEnable = 1;
    InitStatus       = 1;
  (default) -> Init
  Init -> Clear_Error : [ButtonStatus == 1 || ReadError ~= 1]
  Wait -> Init [order 3] : [ReadError ~= 1]
  SetCurrentMode -> Init : [ReadError ~= 1]
  Clear_Error -> Wait : [aux>2000]
  Wait -> Wait [order 1] : [ButtonStatus==0 && ReadError == 1]
  Wait -> SetCurrentMode [order 2] : [ButtonStatus==2 && ReadError == 1]
  data: ButtonStatus input single; ClearError output single; DeviceMode output single; BrakeCtrl output single; ReadError input single; aux2 local single; aux local single; PowerEnable output single; InitStatus output single

== stateflow chart SpeedgoatCANOpen2Buses100us/Trike Application Layer/System_Init/Brakes_DunkMotor_Init/DunkD_Brake_Init_CurrentMode ==
  state Init
    entry:
    ClearError       = 0;
    DeviceMode   = 0;
    BrakeCtrl        = 0;
    PowerEnable = 0;
    aux                 = 0;
    InitStatus        = 0;
  state Clear_Error
    du:
    ClearError = 1;
    aux=aux+1;
    InitStatus = 0;
  state Wait
    en:
    BrakeCtrl = 2;
    aux = 0;
    InitStatus = 0;
  state SetCurrentMode
    du:
    DeviceMode  = 2;
    PowerEnable = 1;
    InitStatus       = 1;
  (default) -> Init
  Init -> Clear_Error : [ButtonStatus == 1 || ReadError ~= 1]
  Wait -> Init [order 3] : [ReadError ~= 1]
  SetCurrentMode -> Init : [ReadError ~= 1]
  Clear_Error -> Wait : [aux>2000]
  Wait -> Wait [order 1] : [ButtonStatus==0 && ReadError == 1]
  Wait -> SetCurrentMode [order 2] : [ButtonStatus==2 && ReadError == 1]
  data: ButtonStatus input single; ClearError output single; DeviceMode output single; BrakeCtrl output single; ReadError input single; aux2 local single; aux local single; PowerEnable output single; InitStatus output single

== stateflow chart SpeedgoatCANOpen2Buses100us/Trike Application Layer/System_Init/EnableCtrl ==
  state Init
    du:
    Enable    =  0;
  state Enable_Control
    du:
    Enable    =  1;
  (default) -> Init
  Init -> Enable_Control : [ButtonStatus == 6 ]
  Enable_Control -> Init : [ButtonStatus == 7 ]
  data: ButtonStatus input single; Enable output single

== matlab function SpeedgoatCANOpen2Buses100us/Trike Application Layer/System_Control/TiltingControl/TiltingController/PID_Adaptiv_V2/PID_ctrl/Subsystem/MATLAB Function ==
  data: gradKi input; Ki output; gradKd input; gradKp input; Kd output; Kp output; alpha input; Kp_old input; Ki_old input; Kd_old input; gradKp_old input; gradKi_old input; gradKd_old input; gradKp_old output; gradKi_old output; gradKd_old output
function [Ki,Kd,Kp,gradKp_old,gradKi_old,gradKd_old] = fcn(gradKi,gradKd,gradKp, alpha, Kp_old, Ki_old, Kd_old,gradKp_old,gradKi_old,gradKd_old)



% v = beta*(oldGrad) + (1-beta)*grad;
% oldGrad = v;
% param = param - alpha*v;
beta = 0.8;
Vkp = beta*gradKp_old + (1-beta)*gradKp;
Vki = beta*gradKi_old + (1-beta)*gradKi;
Vkd = beta*gradKd_old + (1-beta)*gradKd;

Kp = Kp_old - alpha*Vkp;
Ki = Ki_old - alpha*Vki;
Kd = Kd_old - alpha*Vkd;

gradKp_old = Vkp;
gradKi_old = Vki;
gradKd_old = Vkd;


end

== matlab function SpeedgoatCANOpen2Buses100us/Trike Application Layer/System_Control/TiltingControl/TiltingController/PID_Incremental_V2/MATLAB Function ==
  data: PosRef input; LTiltCurrRef output; Pos input; En input; RTiltCurrRef output; c1 output; c2 output
function [LTiltCurrRef, RTiltCurrRef,c1,c2] = fcnb(PosRef,Pos,En)
persistent uk1 ek1 

if (isempty(uk1))
    uk1 = 0;
    ek1 = 0;  
end

% +/- 0.076 m
pos_lim = 0.02;
imax = 10;
   
if En == 0 
    uk1 = 0;
    ek1 = 0;
    Kp = 0;
    
    Kr = Kp;
    Ti = 1e6;    
%   Kd = 0;
else
    
    Kp = 1500;  % 800 pt 1ms
    Ki = 400;     % 5    
%   Kd = 0;     % 5

    Kr = Kp;
    Ti = Kp / Ki;    
end


% Td = Kd / Kp;

Ts = 0.005;

if (PosRef > pos_lim)
    PosRef = pos_lim;
end
if (PosRef <- pos_lim)
   PosRef = -pos_lim;
end

e = PosRef - Pos;

c1 = Kr * (1 + Ts / Ti); % + Td / Ts
c2 = -Kr;                % + 2 * Td / Ts
                         % c3 = - Kr * Td / Ts
Du = c1 * e + c2 * ek1;  % + c3 * ek2
u  = uk1 + Du;

if (u > imax)
    u = imax;
end
if (u<-imax)
    u=-imax;
end

LTiltCurrRef = u;
RTiltCurrRef = - u;

uk1   = u;
ek1   = e;

== matlab function SpeedgoatCANOpen2Buses100us/Trike Application Layer/System_Control/TiltingControl/TiltingController/PID_Adaptiv_V2/PID_ctrl/Subsystem4/MATLAB Function1 ==
  data: u input; y output
function y = fcn(u)
if u == 0
    y = 0.0001;
else
y = u;
end

== matlab function SpeedgoatCANOpen2Buses100us/Trike Application Layer/System_Control/TiltingControl/TiltingController/PID_Adaptiv_V2/PID_ctrl/Subsystem4/derivativeNN ==
  data: X1 input size=[1,1]; X2 input size=[1,1]; dydu output size=[1,1]; Win input size=[20,2]; Wout input size=[1,20]; bin input size=[20,1]

function dydu  = ffnetforcast(X1,X2, Win, Wout, bin)
X = [X1;X2];
netin = Win*X + bin;
dydu_pre = Win'*(Wout'.*hprime(netin));
dydu = dydu_pre(1,1);
function y = hprime(x)
    y = (1-tanh(x).^2);
end
end

== matlab function SpeedgoatCANOpen2Buses100us/Trike Application Layer/System_Control/DirectionControl/P Direction Controller ==
  data: DirectionRef input; SpeedRef output; Direction input
function SpeedRef  = fcn(DirectionRef,Direction)


if (DirectionRef>90)
    DirectionRef=90;
end
if (DirectionRef<-90)
    DirectionRef=-90;
end
err = DirectionRef - Direction;

Kp = 70;

SpeedRef = Kp * err;  


end

== matlab function SpeedgoatCANOpen2Buses100us/Trike Application Layer/System_Control/TiltingControl/TiltingController/PID_Incremental_V1/PI_incremental Tilting Controller ==
  data: PosRef input; LTiltCurrRef output; Pos input; RTiltCurrRef output; En input; up output; ui output; ud output
function [LTiltCurrRef, RTiltCurrRef,up,ui,ud] = fcn(PosRef,Pos,En)
persistent uk1 ek1 udk1 Posk1
if (isempty(uk1))
    Posk1 = 0;
    udk1 = 0;
    uk1 = 0;
    ek1 = 0; 
end

% +/- 0.076 m
pos_lim = 0.02;
imax = 10;


if En == 0
    
    u = 0;
    Kp = 0;
    Ki = 0;
    Kd = 0;
else
    
    Kp = 1200;  % 800 pt 1ms
    Ki = 3;     % 5
    Kd = 2;     % 5
    
end


if (PosRef > pos_lim)
    PosRef = pos_lim;
end
if (PosRef <- pos_lim)
   PosRef = -pos_lim;
end

e = PosRef - Pos;

Te = 0.005;
up = Kp * (e - ek1);
ui = Ki * e;
ud = -udk1 - Kd * (Pos - Posk1)*2/Te;


Du = up + ui + ud;

u = uk1 + Du;

if (u > imax)
    u = imax;
end
if (u<-imax)
    u=-imax;
end

LTiltCurrRef =  u;
RTiltCurrRef = -u;

Posk1 = Pos;
udk1  = ud;
uk1   = u;
ek1   = e;

== matlab function SpeedgoatCANOpen2Buses100us/Trike Application Layer/System_Control/TiltingControl/ServoTilting ==
  data: SteerAngle input; TravelingSpeed input; TiltingAngle output
function TiltingAngle  = CalcTiltAngle(SteerAngle,TravelingSpeed)
%SteerAngle [rad]
%TravelingSpeed [m/s]
L = 1.025;
g = 9.81;
TiltingAngle = atan(TravelingSpeed^2/(L*g)*sin(SteerAngle));
TiltingAngle = TiltingAngle *180/pi;
% TiltingAngle [deg]

== stateflow chart SpeedgoatCANOpen2Buses100us/Trike Application Layer/System_Init/Steering_DunkMotor_Init/DunkA_Steering_Init_SpeedMode ==
  state Init
    entry:
    ClearError       = 0;
    DeviceMode   = 0;
    BrakeCtrl        = 0;
    PowerEnable = 0;
    aux                 = 0;
    InitStatus        = 0;
  state Clear_Error
    du:
    ClearError = 1;
    aux=aux+1;
    InitStatus = 0;
  state Wait
    en:
    BrakeCtrl = 2;
    aux = 0;
    InitStatus = 0;
  state SetCurrentMode
    du:
    DeviceMode  = 3; % SpeedMode
    PowerEnable = 1;
    InitStatus       = 1;
  (default) -> Init
  Init -> Clear_Error : [ButtonStatus == 1 || ReadError ~= 1]
  Wait -> Init [order 3] : [ReadError ~= 1]
  SetCurrentMode -> Init : [ReadError ~= 1]
  Clear_Error -> Wait : [aux>2000]
  Wait -> Wait [order 1] : [ButtonStatus==0 && ReadError == 1]
  Wait -> SetCurrentMode [order 2] : [ButtonStatus==2 && ReadError == 1]
  data: ButtonStatus input single; ClearError output single; DeviceMode output single; BrakeCtrl output single; ReadError input single; aux2 local single; aux local single; PowerEnable output single; InitStatus output single

== matlab function SpeedgoatCANOpen2Buses100us/Trike Application Layer/System_Init/MATLAB Function ==
  data: ButtonStatus input; button output
function button = JoystickButtonStatus(ButtonStatus)
aux = 0;
switch (ButtonStatus)
    case 1
        aux = 1;
    case 2
        aux = 2;
    case 4
        aux = 3;
    case 8
        aux = 4;
    case 16
        aux = 5;
    case 32
        aux = 6; 
    case 64
        aux = 7;
    case 128 
        aux = 8;
    otherwise
        aux = 0;
end
button =aux;

== matlab function SpeedgoatCANOpen2Buses100us/Trike Application Layer/Subsystem1/HeartBeatgenerator ==
  data: HB output
function HB = HBGenerator
persistent tact Heartbeat
if (isempty(Heartbeat))
    Heartbeat = 0;
    tact = 0;
end
tact=tact+1;
if (tact>10)
    tact=0;
    Heartbeat=Heartbeat+1;
    if (Heartbeat>127)
        Heartbeat = 0;    
    end
end
HB = Heartbeat;

== matlab function SpeedgoatCANOpen2Buses100us/Trike Application Layer/System_Init/MATLAB Function1 ==
  data: ButtonStatus input; Byte0 output; LongCmd input
function Byte0 = TractionCtrl(ButtonStatus, LongCmd)
Direction =0;
if (ButtonStatus==8)
    if(LongCmd>0)
        Direction = 4;
    elseif (LongCmd<0)
        Direction = 8;
    end
 end
Byte0 =160+Direction;
